simulink subsystem "NoSuspensionFront"  (R2024a)
settings: Solver=VariableStepAuto  StartTime=0.0  StopTime=10.0  RelTol=1e-3
undefined symbols (not defined in the file): PlntWhlNumFrnt
settings Model: ModifiedByFormat=The MathWorks, Inc.  Creator=The MathWorks, Inc.  LastModifiedBy=The MathWorks, Inc.
settings DebuggingCC: SubsystemReferenceDiagnosticForUnitTest=warning
settings RTWCC: GPUComputeCapability=3.5

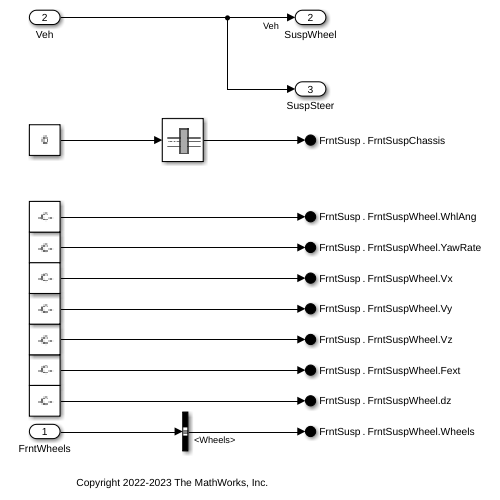
[thumbnail: Simulink's stored preview of the top-level diagram]
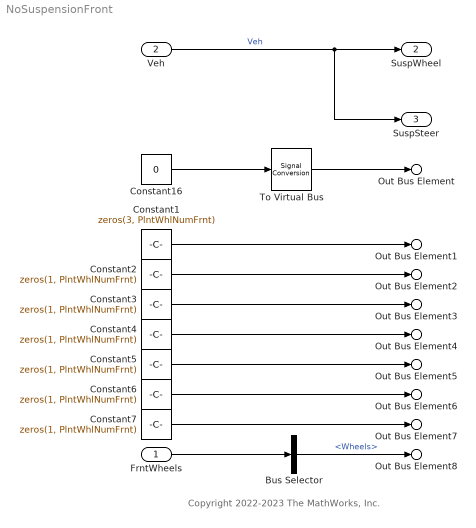
== system NoSuspensionFront ==
  note: Copyright 2022-2023 The MathWorks, Inc.
  FrntWheels : Inport
  Veh : Inport  Port=2
  Bus Selector : BusSelector  OutputSignals=Wheels
  Constant1 : Constant  Value=zeros(3, PlntWhlNumFrnt)  SampleTime=Inf
  Constant16 : Constant  Value=0  OutDataTypeStr=Bus: FrntSuspChassisBUS  SampleTime=Inf
  Constant{2..7} (6 alike) : Constant  Value=zeros(1, PlntWhlNumFrnt)  SampleTime=Inf
  To Virtual Bus : SignalConversion  ConversionOutput=Virtual bus  OverrideOpt=off
  Out Bus Element : Outport  PortName=FrntSusp  Element=FrntSuspChassis
  Out Bus Element1 : Outport  PortName=FrntSusp  Element=FrntSuspWheel.WhlAng
  Out Bus Element2 : Outport  PortName=FrntSusp  Element=FrntSuspWheel.YawRate
  Out Bus Element3 : Outport  PortName=FrntSusp  Element=FrntSuspWheel.Vx
  Out Bus Element4 : Outport  PortName=FrntSusp  Element=FrntSuspWheel.Vy
  Out Bus Element5 : Outport  PortName=FrntSusp  Element=FrntSuspWheel.Vz
  Out Bus Element6 : Outport  PortName=FrntSusp  Element=FrntSuspWheel.Fext
  Out Bus Element7 : Outport  PortName=FrntSusp  Element=FrntSuspWheel.dz
  Out Bus Element8 : Outport  PortName=FrntSusp  Element=FrntSuspWheel.Wheels
  SuspWheel : Outport  Port=2
  SuspSteer : Outport  Port=3
  wires:
  Bus Selector/1 -> Out Bus Element8/1  "<Wheels>"
  FrntWheels/1 -> Bus Selector/1
  Constant7/1 -> Out Bus Element7/1
  Constant6/1 -> Out Bus Element6/1
  Constant5/1 -> Out Bus Element5/1
  Constant4/1 -> Out Bus Element4/1
  Constant3/1 -> Out Bus Element3/1
  Constant2/1 -> Out Bus Element2/1
  Constant1/1 -> Out Bus Element1/1
  Veh/1 -> SuspWheel/1, SuspSteer/1  "Veh"
  To Virtual Bus/1 -> Out Bus Element/1
  Constant16/1 -> To Virtual Bus/1
